simulink model "UKF_new"  (R2021a)
settings: Solver=VariableStepAuto  StartTime=0.0  StopTime=120002  RelTol=1e-3
values from neighbouring files (symbols this model uses):
  Ro = 70.6*1e-3    (= 0.0706)    [myMeasurementFcn.m]
undefined symbols (not defined in the file or in its folder): A, B, C, CN, D, Discrete, eta, Rp, Rs, tau_p, tau_s, Time, ts
libraries: simulink x5, ctrlSharedLib x1, sharedTrackingLibrary x1
settings Model: Creator=Angga  LastModifiedBy=Angga

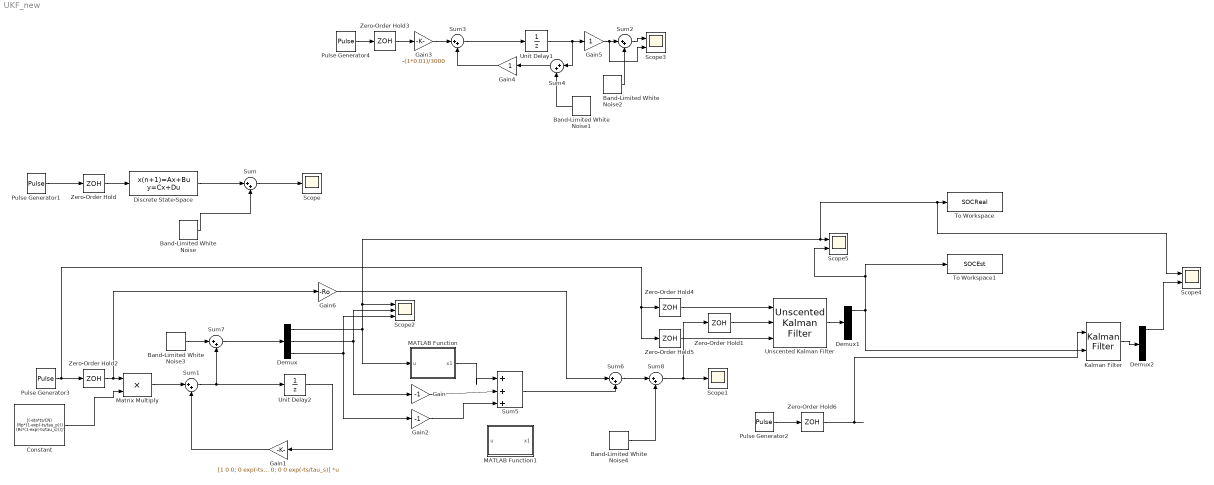
== system UKF_new ==
  Band-Limited White Noise : simulink/Sources/Band-Limited White Noise  Cov=[1e-6]  Ts=1  seed=[23341]
  Band-Limited White Noise1 : simulink/Sources/Band-Limited White Noise  Cov=[1e-8]  Ts=1  seed=[23341]
  Band-Limited White Noise2 : simulink/Sources/Band-Limited White Noise  Cov=[1e-8]  Ts=1  seed=[23341]
  Band-Limited White Noise3 : simulink/Sources/Band-Limited White Noise  Cov=[1e-8]  Ts=1  seed=[23341]
  Band-Limited White Noise4 : simulink/Sources/Band-Limited White Noise  Cov=[0.1]  Ts=1  seed=[23341]
  Constant : Constant  Value=[(-eta*ts/CN) (Rp*(1-exp(-ts/tau_p))) (Rs*(1-exp(-ts/tau_s)))]'
  Demux : Demux  Outputs=3
  Demux1 : Demux  Outputs=3
  Demux2 : Demux
  Discrete State-Space : DiscreteStateSpace  B=-(1*0.01)/3000  D=0  InitialCondition=1
  Gain : Gain  Gain=-1
  Gain1 : Gain  Gain=[1 0 0; 0 exp(-ts/tau_p) 0; 0 0 exp(-ts/tau_s)]  Multiplication=Matrix(K*u) (u vector)
  Gain2 : Gain  Gain=-1
  Gain3 : Gain  Gain=-(1*0.01)/3000
  Gain4 : Gain
  Gain5 : Gain
  Gain6 : Gain  Gain=-Ro
  Kalman Filter : ctrlSharedLib/Kalman Filter  TimeDomain=Discrete-Time  UseCurrentEstimator=on  ModelSource=Individual A, B, C, D matrices  ModelSourceVariable=ss(0.95,1,1,0,1)  A=A  B=B  C=C  D=D  NumberOfStates=1  NumberOfInputs=1  NumberOfOutputs=1  InitialEstimateSource=Dialog  X0=[0 0 0 1]'  P0=10  UseK=off  UseGH=off  NumberOfProcessNoiseInputs=1  G=1  TimeInvariantG=on  H=0  TimeInvariantH=on  Q="diag([1e-8 1e-8 1e-8  0])"  TimeInvariantQ=on  R=0.1  TimeInvariantR=on  N=0  TimeInvariantN=on  AddInputPort=on  AddEnablePort=off  OutputEstimatedY=off  OutputP=off  Ts=1
  MATLAB Function : MATLAB Function  TreatAsAtomicUnit=on
  MATLAB Function1 : MATLAB Function  TreatAsAtomicUnit=on
  Matrix Multiply : Product
  Pulse Generator{1..4} (4 alike) : DiscretePulseGenerator  PulseType=Time based  Amplitude=25  Period=5000  PulseWidth=10
  Scope : Scope
  Scope1 : Scope
  Scope2 : Scope  NumInputPorts=3
  Scope3 : Scope  NumInputPorts=2
  Scope4 : Scope  NumInputPorts=2
  Scope5 : Scope  NumInputPorts=2
  Sum{,1..4,6..8} (8 alike) : Sum  Inputs=|++
  Sum5 : Sum  Inputs=|+++
  To Workspace : ToWorkspace  VariableName=SOCReal  SampleTime=-1
  To Workspace1 : ToWorkspace  VariableName=SOCEst  SampleTime=-1
  Unit Delay1 : UnitDelay  InitialCondition=1  HasFrameUpgradeWarning=on
  Unit Delay2 : UnitDelay  InitialCondition=[1 0 0]'  HasFrameUpgradeWarning=on
  Unscented Kalman Filter : sharedTrackingLibrary/Unscented Kalman Filter  StateTransitionFcn=myStateTransitionFcn  HasAdditiveProcessNoise=Additive  ProcessNoise=diag([1e-8 1e-8 1e-8])  HasTimeVaryingProcessNoise=off  HasStateTransitionFcnExtraArgument=1  InitialState=[0.99 0 0]'  InitialStateCovariance=0.1*eye(3)  Alpha=1e-3  Beta=2  Kappa=0  MeasurementFcn1=myMeasurementFcn  HasMeasurementEnablePort1=off  HasAdditiveMeasurementNoise1=Additive  MeasurementNoise1=0.1  HasTimeVaryingMeasurementNoise1=off  HasMeasurementFcnExtraArgument1=1  MeasurementFcn2=myMeasurementFcn  HasMeasurementEnablePort2=off  HasAdditiveMeasurementNoise2=Additive  MeasurementNoise2=1  HasTimeVaryingMeasurementNoise2=off  HasMeasurementFcnExtraArgument2=0  MeasurementFcn3=myMeasurementFcn  HasMeasurementEnablePort3=off  HasAdditiveMeasurementNoise3=Additive  MeasurementNoise3=1  HasTimeVaryingMeasurementNoise3=off  HasMeasurementFcnExtraArgument3=0  MeasurementFcn4=myMeasurementFcn  HasMeasurementEnablePort4=off  HasAdditiveMeasurementNoise4=Additive  MeasurementNoise4=1  HasTimeVaryingMeasurementNoise4=off  HasMeasurementFcnExtraArgument4=0  MeasurementFcn5=myMeasurementFcn  HasMeasurementEnablePort5=off  HasAdditiveMeasurementNoise5=Additive  MeasurementNoise5=1  HasTimeVaryingMeasurementNoise5=off  HasMeasurementFcnExtraArgument5=0  EnableMultirate=off  StateTransitionFcnSampleTime=1  MeasurementFcn1SampleTime=1  MeasurementFcn2SampleTime=1  MeasurementFcn3SampleTime=1  MeasurementFcn4SampleTime=1  MeasurementFcn5SampleTime=1  UseCurrentEstimator=on  OutputStateCovariance=off  DataType=double  SampleTime=1  NumberOfMeasurements=1
      settings: SourceProductBaseCode=CT,DR,TF,ID,LP,NV,AR,RO,RR,UV,VE
  Zero-Order Hold{,1..6} (7 alike) : ZeroOrderHold
  wires:
  Pulse Generator1/1 -> Zero-Order Hold/1
  Zero-Order Hold/1 -> Discrete State-Space/1
  Band-Limited White Noise/1 -> Sum/2
  Discrete State-Space/1 -> Sum/1
  Sum/1 -> Scope/1
  Pulse Generator3/1 -> Zero-Order Hold4/1, Zero-Order Hold5/1, Zero-Order Hold2/1
  Zero-Order Hold2/1 -> Gain6/1, Matrix Multiply/1
  Constant/1 -> Matrix Multiply/2
  Matrix Multiply/1 -> Sum1/1
  Gain3/1 -> Sum3/1
  Sum2/1 -> Scope3/1
  Gain5/1 -> Scope3/2, Sum2/1
  Gain4/1 -> Sum3/2
  Sum4/1 -> Gain4/1
  Sum3/1 -> Unit Delay1/1
  Unit Delay1/1 -> Sum4/1, Gain5/1
  Zero-Order Hold3/1 -> Gain3/1
  Band-Limited White Noise1/1 -> Sum4/2
  Band-Limited White Noise2/1 -> Sum2/2
  Pulse Generator4/1 -> Zero-Order Hold3/1
  Sum1/1 -> Unit Delay2/1, Sum7/2
  Unit Delay2/1 -> Gain1/1
  Gain1/1 -> Sum1/2
  Demux/1 -> Scope2/1, Scope4/1, To Workspace/1, Scope5/1, MATLAB Function/1(u)
  MATLAB Function/1(x1) -> Sum5/1
  Demux/2 -> Scope2/2, Gain/1
  Gain/1 -> Sum5/2
  Demux/3 -> Scope2/3, Gain2/1
  Gain2/1 -> Sum5/3
  Sum5/1 -> Sum6/2
  Gain6/1 -> Sum6/1
  Band-Limited White Noise3/1 -> Sum7/1
  Sum7/1 -> Demux/1
  Sum6/1 -> Sum8/1
  Band-Limited White Noise4/1 -> Sum8/2
  Sum8/1 -> Zero-Order Hold1/1, Scope1/1
  Unscented Kalman Filter/1 -> Demux1/1
  Zero-Order Hold1/1 -> Unscented Kalman Filter/2
  Zero-Order Hold4/1 -> Unscented Kalman Filter/1
  Zero-Order Hold5/1 -> Unscented Kalman Filter/3
  Demux1/1 -> Kalman Filter/2, To Workspace1/1, Scope5/2
  Pulse Generator2/1 -> Zero-Order Hold6/1
  Zero-Order Hold6/1 -> Kalman Filter/1
  ? -> ?
  Kalman Filter/1 -> Demux2/1
  Demux2/1 -> Scope4/2

== matlab function UKF_new/MATLAB Function ==
  data: u input; x1 output
function x1 = fcn(u)

x1 = 3.8194*u^6 - 4.6554*u^5 - 8.9009*u^4 + 19.3256*u^3 - 11.9564*u^2 + 3.291*u + 3.2518;
end

== matlab function UKF_new/MATLAB Function1 ==
  data: u input; x1 output
function x1 = fcn(u)

x1 = 0.7428*u+3.3613;
end
